simulink model "STank_01"  (R2013a)
settings: Solver=ode45  StartTime=0.0  StopTime=1000  RelTol=1e-3
settings Model: Creator=Cristhian Ivan  LastModifiedBy=Cristhian Ivan
settings DataIOCC: SignalLoggingSaveFormat=ModelDataLogs
settings OptimizationCC: InitFltsAndDblsToZero=on
settings DebuggingCC: SaveWithParameterizedLinksMsg=none  SignalResolutionControl=TryResolveAllWithWarning  MultiTaskDSMMsg=warning  MultiTaskCondExecSysMsg=none  StrictBusMsg=None
settings RTWCC: IncludeERTFirstTime=on
settings GRTTargetCC: TargetFcnLib=ansi_tfl_tmw.mat  CombineOutputUpdateFcns=off  GRTInterface=on

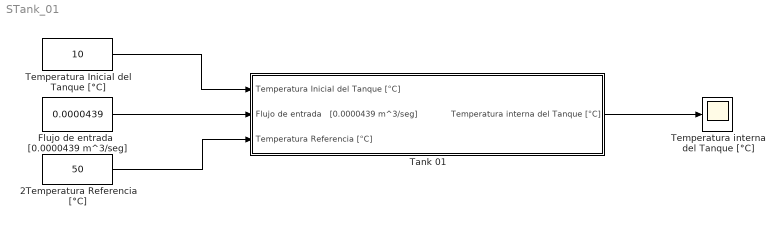
== system STank_01 ==
  2Temperatura Referencia [°C] : Constant  Value=50
  "Flujo de entrada   [0.0000439 m^3/seg] " : Constant  Value=0.0000439
  Tank 01 : Subsystem
  Temperatura Inicial del Tanque [°C] : Constant  Value=10
  Temperatura interna del Tanque [°C] : Scope
      settings: TimeRange=10  YMin=20  YMax=45
  wires:
  Temperatura Inicial del Tanque [°C]/1 -> Tank 01/1(Temperatura Inicial del Tanque [°C])
  "Flujo de entrada   [0.0000439 m^3/seg] "/1 -> Tank 01/2(Flujo de entrada   [0.0000439 m^3/seg])
  2Temperatura Referencia [°C]/1 -> Tank 01/3(Temperatura Referencia [°C])
  Tank 01/1(Temperatura interna del Tanque [°C]) -> Temperatura interna del Tanque [°C]/1

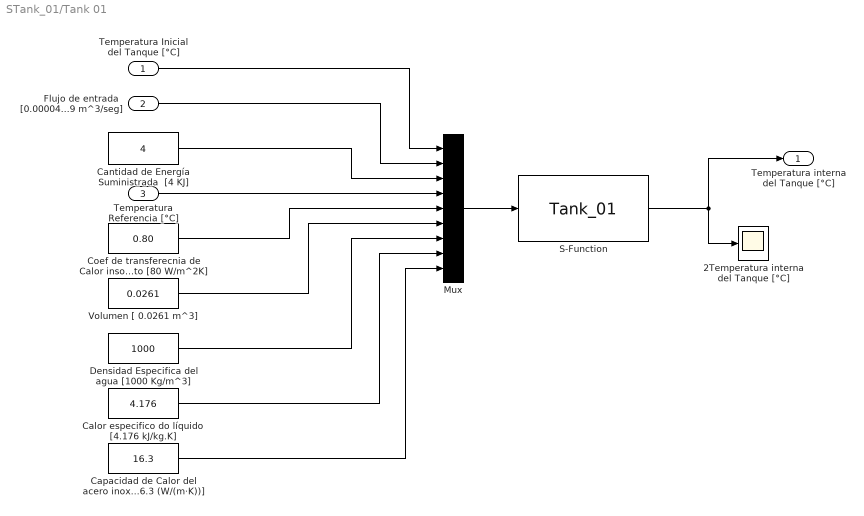
== system STank_01/Tank 01 ==
  Temperatura Inicial del Tanque [°C] : Inport
  Flujo de entrada   [0.0000439 m^3/seg] : Inport  Port=2
  Temperatura Referencia [°C] : Inport  Port=3
  2Temperatura interna del Tanque [°C] : Scope
      settings: TimeRange=10  YMin=20  YMax=45
  Calor especifico do líquido  [4.176 kJ/kg.K] : Constant  Value=4.176
  Cantidad de Energía Suministrada  [4 KJ] : Constant  Value=4
  Capacidad de Calor del acero inox [16.3 (W/(m·K))] : Constant  Value=16.3
  Coef de transferecnia de Calor insolamiento [80 W/m^2K] : Constant  Value=0.80
  Densidad Especifica del agua [1000 Kg/m^3] : Constant  Value=1000
  Mux : Mux  Inputs=9
  S-Function : S-Function  FunctionName=Tank_01  EnableBusSupport=off
  Volumen [ 0.0261 m^3] : Constant  Value=0.0261
  Temperatura interna del Tanque [°C] : Outport
  wires:
  Cantidad de Energía Suministrada  [4 KJ]/1 -> Mux/3
  Volumen [ 0.0261 m^3]/1 -> Mux/6
  Capacidad de Calor del acero inox [16.3 (W/(m·K))]/1 -> Mux/9
  Calor especifico do líquido  [4.176 kJ/kg.K]/1 -> Mux/8
  S-Function/1 -> Temperatura interna del Tanque [°C]/1, 2Temperatura interna del Tanque [°C]/1
  Coef de transferecnia de Calor insolamiento [80 W/m^2K]/1 -> Mux/5
  Mux/1 -> S-Function/1
  Densidad Especifica del agua [1000 Kg/m^3]/1 -> Mux/7
  Temperatura Inicial del Tanque [°C]/1 -> Mux/1
  Flujo de entrada   [0.0000439 m^3/seg]/1 -> Mux/2
  Temperatura Referencia [°C]/1 -> Mux/4
